simulink model "s_ss"  (R2013a)
settings: Solver=ode45  StartTime=0.0  StopTime=10.0  RelTol=1e-3
undefined symbols (not defined in the file or in its folder): KD, KI, Kp
settings Model: Creator=mainster  LastModifiedBy=mainster

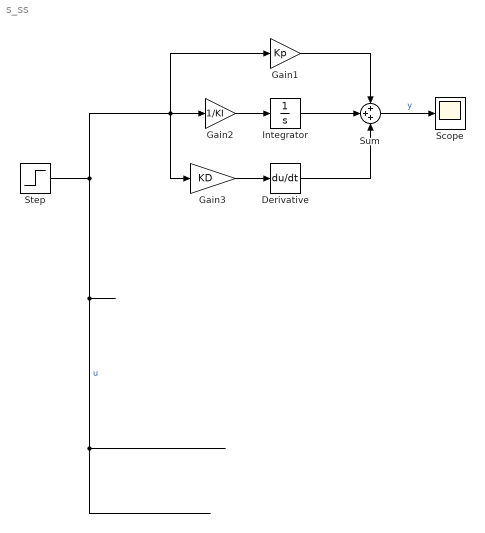
== system s_ss ==
  Derivative : Derivative
  Gain1 : Gain  Gain=Kp
  Gain2 : Gain  Gain=1/KI
  Gain3 : Gain  Gain=KD
  Integrator : Integrator
  Scope : Scope
  Step : Step  Time=10e-3  SampleTime=0
  Sum : Sum  Inputs=+++
  wires:
  Step/1 -> Gain1/1, Gain3/1, Gain2/1  "u"
  Gain1/1 -> Sum/1
  Integrator/1 -> Sum/2
  Gain3/1 -> Derivative/1
  Derivative/1 -> Sum/3
  Gain2/1 -> Integrator/1
  Sum/1 -> Scope/1  "y"
